simulink model "gm_sampleModel1714_sub"  (R2023a)
settings: Solver=VariableStepAuto  StartTime=0.0  StopTime=10.0  RelTol=1e-3
libraries: simulink x2, hdlsllib x1
settings Model: Creator=user1  LastModifiedBy=user1
settings OptimizationCC: BlockReduction=off  ConditionallyExecuteInputs=off
settings DebuggingCC: InheritedTsInSrcMsg=none

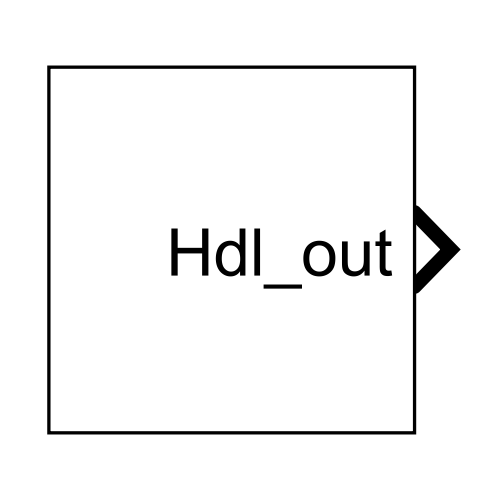
[thumbnail: Simulink's stored preview of the top-level diagram]
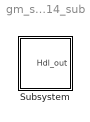
== system gm_sampleModel1714_sub ==
  Subsystem : Subsystem

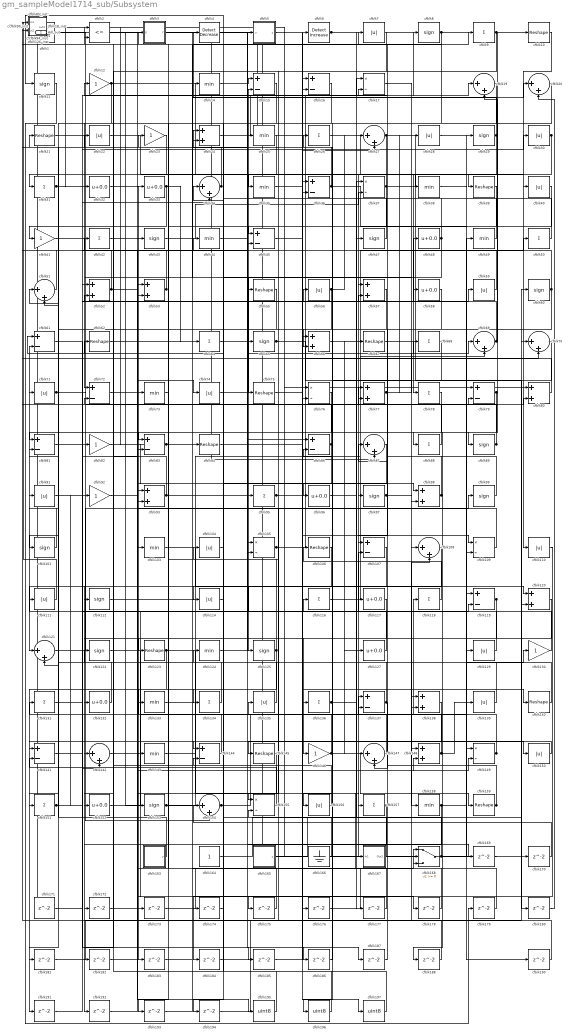
== system gm_sampleModel1714_sub/Subsystem ==
  cfblk1 : hdlsllib/Logic and Bit Operations/Bit Shift  mode=Shift Left Logical  N=0
  cfblk{10,21,39,55,62,67,75,84,106,123,140,145,159} (13 alike) : Reshape
  cfblk{8,11,29,43,47,60,65,89,97,99,101,112,122,125,153} (15 alike) : Signum
  cfblk102_inst : Subsystem
  cfblk{14,25,35,38,44,49,73,103,124,133,143,158} (12 alike) : MinMax  OutDataTypeStr=uint8
  cfblk{7,22,28,30,40,56,59,71,74,91,104,110..111,114,129,135,139,150,156} (19 alike) : Abs  OutDataTypeStr=uint8  SaturateOnIntegerOverflow=off
  cfblk{17,37,76,105,109,149,155} (7 alike) : Product  Inputs=*/  OutDataTypeStr=uint8  RndMeth=Zero  SaturateOnIntegerOverflow=on
  cfblk{15..16,36,45,61,72,79,81,83,86,107,119,137,141,144} (15 alike) : Sum  Inputs=+-  OutDataTypeStr=uint8
  cfblk{19..20,27,34,51,69..70,87,108,121,142,147,154} (13 alike) : Sum  Inputs=|++  OutDataTypeStr=uint8
  cfblk113_inst : Subsystem
  cfblk{9,26,31,42,50,64,68,78,88,95,116,118,131,134,136,151,157} (17 alike) : Sum  Inputs=+  OutDataTypeStr=uint8
  cfblk{32..33,48,58,96,117,127,132,152} (9 alike) : Bias  Bias=0.0  SaturateOnIntegerOverflow=off
  cfblk{12,23,41,82,92,130,146} (7 alike) : Gain  OutDataTypeStr=uint8
  cfblk{24,52..53,57,66,77,80,93,98,120,138,148} (12 alike) : Sum  OutDataTypeStr=uint8
  cfblk126_inst : Subsystem
  cfblk128_inst : Subsystem
  cfblk163 : Subsystem  mask(Counter Free-Running){NumBits=double(16), tsamp=double(-1)}
      mask prompts: NumBits "Simulink:masks:NumberOfBits_MP"; tsamp "Simulink:masks:SampleTime_MP"
      mask help: Simulink:masks:CounterFreeRunning_MD
  cfblk164 : Constant  OutDataTypeStr=uint8  SampleTime=-1
  cfblk165 : Subsystem  mask(Counter Limited){uplimit=double(7), tsamp=double(-1)}
      mask prompts: uplimit "Simulink:masks:UpperLimit_MP"; tsamp "Simulink:masks:SampleTime_MP"
      mask help: Simulink:masks:CounterLimited_MD
      mask init:
      | nbits = double(8);
      | tsamp = double(-1);
      | uplimit = double(7);
  cfblk166 : Ground
  cfblk167 : Subsystem
  cfblk168 : Switch  OutDataTypeStr=uint8  SaturateOnIntegerOverflow=off  InputSameDT=off
  cfblk{169..188,190..194} (25 alike) : Delay  SampleTime=1
  cfblk18_inst : Subsystem
  cfblk195 : DataTypeConversion  OutDataTypeStr=uint8  SaturateOnIntegerOverflow=off  RndMeth=Floor
  cfblk196 : DataTypeConversion  OutDataTypeStr=uint8  SaturateOnIntegerOverflow=off  RndMeth=Floor
  cfblk197 : DataTypeConversion  OutDataTypeStr=uint8  SaturateOnIntegerOverflow=off  RndMeth=Floor
  cfblk2 : RelationalOperator  Operator=<=  OutDataTypeStr=boolean  InputSameDT=off
  cfblk3 : Subsystem  mask(Detect Fall Nonpositive){vinit=double(0), InputProcessing=Elements as channels (sample based), OutDataTypeStr=uint8}
      mask prompts: vinit "Simulink:masks:InitialCondition_MP"; InputProcessing "Simulink:masks:InputProcessing_MP"; OutDataTypeStr "Simulink:masks:OutputDataType_MP"
      mask help: Simulink:masks:DetectFallNonpositive_MD
      mask init:
      | InputProcessing = 'Elements as channels (sample based)';
      | OutDataTypeStr = 'uint8';
      | vinit = double(0);
      mask TypeOptions InputProcessing: Simulink:masks:ColumnsAsChannelsFrameBased | Simulink:masks:ElementsAsChannelsSampleBased
      mask TypeOptions OutDataTypeStr: Simulink:masks:uint8 | Simulink:masks:boolean
      mask Display: fprintf('U <= 0\n&  NOT\nU/z <= 0')
  cfblk4 : simulink/Logic and Bit Operations/Detect Decrease  vinit=0.0  OutDataTypeStr=uint8
      settings: LibrarySourceBlock=|
      | hdlsllib/Logic and Bit
      | Operations/Detect
      | Decrease
  cfblk5 : Subsystem  mask(Compare To Constant){relop=<=, const=double(3), OutDataTypeStr=uint8, ZeroCross=on}
      mask prompts: relop "Simulink:masks:Operator_MP"; const "Simulink:masks:ConstantValue_MP"; OutDataTypeStr "Simulink:masks:OutputDataType_MP"; ZeroCross "Simulink:masks:EnableZerocrossingDetection_MP"
      mask help: Simulink:masks:CompareToConstant_MD
      mask init:
      | OutDataTypeStr = 'uint8';
      | ZeroCross = 'on';
      | blkName = 'sampleModel1714_sub/Subsystem/cfblk5';
      | const = double(3);
      | const_str = '3.0';
      | const_val = double(3);
      | relop = '<=';
      | setValue = 'fixdt(0, 8)';
      | str = '<= 3';
      mask TypeOptions relop: == | ~= | < | <= | >= | >
      mask TypeOptions OutDataTypeStr: Simulink:masks:uint8 | Simulink:masks:boolean
      mask Callback ZeroCross: sl('zeroCrossEnable', gcbh);
      mask Display: disp(str)
  cfblk6 : simulink/Logic and Bit Operations/Detect Increase  vinit=0.0  OutDataTypeStr=uint8
      settings: LibrarySourceBlock=|
      | hdlsllib/Logic and Bit
      | Operations/Detect
      | Increase
  cfblk85_inst : Subsystem
  cfblk90_inst : Subsystem
  cfblk94_inst : Subsystem
  Hdl_out : Outport  OutDataTypeStr=uint8  SampleTime=1
  wires:
  cfblk1/1 -> cfblk154/2
  cfblk10/1 -> cfblk110/1
  cfblk101/1 -> cfblk61/2
  cfblk102_inst/1(out1) -> cfblk84/1
  cfblk103/1 -> cfblk120/1
  cfblk104/1 -> cfblk11/1
  cfblk105/1 -> cfblk80/2, cfblk19/1
  cfblk106/1 -> cfblk192/1
  cfblk107/1 -> cfblk121/1
  cfblk108/1 -> cfblk125/1
  cfblk109/1 -> cfblk33/1
  cfblk11/1 -> cfblk179/1
  cfblk110/1 -> cfblk184/1
  cfblk111/1 -> cfblk126_inst/1(in1)
  cfblk112/1 -> cfblk50/1
  cfblk113_inst/1(out1) -> cfblk87/2, cfblk128_inst/1(in1)
  cfblk114/1 -> cfblk34/1
  cfblk116/1 -> cfblk69/2
  cfblk117/1 -> cfblk146/1
  cfblk118/1 -> cfblk106/1
  cfblk119/1 -> cfblk142/1, cfblk132/1
  cfblk12/1 -> cfblk72/1, cfblk167/1(In1)
  cfblk120/1 -> cfblk136/1
  cfblk121/1 -> cfblk99/1
  cfblk122/1 -> cfblk175/1
  cfblk123/1 -> cfblk168/1, cfblk191/1
  cfblk124/1 -> cfblk86/1
  cfblk125/1 -> cfblk183/1, cfblk3/1(U)
  cfblk126_inst/1(out1) -> cfblk80/1
  cfblk127/1 -> cfblk107/2
  cfblk128_inst/1(out1) -> cfblk171/1
  cfblk129/1 -> cfblk71/1
  cfblk130/1 -> cfblk15/2
  cfblk131/1 -> cfblk116/1
  cfblk132/1 -> cfblk21/1
  cfblk133/1 -> cfblk5/1(u)
  cfblk134/1 -> cfblk81/2
  cfblk135/1 -> cfblk91/1
  cfblk136/1 -> cfblk47/1, cfblk127/1
  cfblk137/1 -> cfblk147/2, cfblk122/1
  cfblk138/1 -> cfblk152/1
  cfblk139/1 -> cfblk87/1
  cfblk14/1 -> cfblk15/1
  cfblk140/1 -> cfblk111/1
  cfblk141/1 -> cfblk30/1
  cfblk142/1 -> cfblk117/1
  cfblk143/1 -> cfblk76/1
  cfblk144/1 -> cfblk52/2
  cfblk145/1 -> cfblk193/1
  cfblk146/1 -> cfblk93/2, cfblk67/1, cfblk159/1
  cfblk147/1 -> cfblk26/1
  cfblk148/1 -> cfblk139/1, cfblk121/2, cfblk95/1
  cfblk149/1 -> cfblk135/1, cfblk118/1, cfblk131/1
  cfblk15/1 -> cfblk134/1
  cfblk150/1 -> cfblk141/1
  cfblk151/1 -> cfblk56/1, cfblk92/1, cfblk17/2
  cfblk152/1 -> cfblk137/1
  cfblk153/1 -> cfblk148/2, cfblk49/1
  cfblk154/1 -> cfblk16/2, Hdl_out/1
  cfblk155/1 -> cfblk141/2
  cfblk156/1 -> cfblk18_inst/1(in1)
  cfblk157/1 -> cfblk173/1, cfblk172/1
  cfblk158/1 -> cfblk194/1, cfblk130/1
  cfblk159/1 -> cfblk85_inst/2(in2), cfblk52/1
  cfblk16/1 -> cfblk153/1
  cfblk163/1(y) -> cfblk51/1
  cfblk164/1 -> cfblk70/1
  cfblk165/1(y) -> cfblk37/1
  cfblk166/1 -> cfblk105/1
  cfblk167/1(Out1) -> cfblk61/1
  cfblk168/1 -> cfblk79/1, cfblk124/1
  cfblk169/1 -> cfblk1/1
  cfblk17/1 -> cfblk148/1
  cfblk170/1 -> cfblk154/1
  cfblk171/1 -> cfblk34/2
  cfblk172/1 -> cfblk45/2
  cfblk173/1 -> cfblk168/2
  cfblk174/1 -> cfblk144/2
  cfblk175/1 -> cfblk24/1
  cfblk176/1 -> cfblk138/1
  cfblk177/1 -> cfblk93/1
  cfblk178/1 -> cfblk16/1
  cfblk179/1 -> cfblk53/1
  cfblk18_inst/1(out1) -> cfblk29/1
  cfblk180/1 -> cfblk20/2
  cfblk181/1 -> cfblk108/2
  cfblk182/1 -> cfblk119/2
  cfblk183/1 -> cfblk168/3
  cfblk184/1 -> cfblk120/2
  cfblk185/1 -> cfblk36/1
  cfblk186/1 -> cfblk86/2
  cfblk187/1 -> cfblk137/2
  cfblk188/1 -> cfblk155/2
  cfblk19/1 -> cfblk41/1
  cfblk190/1 -> cfblk102_inst/2(in2)
  cfblk191/1 -> cfblk142/2
  cfblk192/1 -> cfblk149/2
  cfblk193/1 -> cfblk9/1
  cfblk194/1 -> cfblk60/1
  cfblk195/1 -> cfblk104/1
  cfblk196/1 -> cfblk2/1
  cfblk197/1 -> cfblk2/2
  cfblk2/1 -> cfblk195/1
  cfblk20/1 -> cfblk123/1
  cfblk21/1 -> cfblk75/1
  cfblk22/1 -> cfblk78/1
  cfblk23/1 -> cfblk53/2
  cfblk24/1 -> cfblk8/1
  cfblk25/1 -> cfblk143/1
  cfblk26/1 -> cfblk39/1
  cfblk27/1 -> cfblk181/1, cfblk180/1
  cfblk28/1 -> cfblk190/1
  cfblk29/1 -> cfblk182/1, cfblk4/1
  cfblk3/1(Y) -> cfblk57/1
  cfblk30/1 -> cfblk36/2, cfblk31/1
  cfblk31/1 -> cfblk108/1, cfblk176/1
  cfblk32/1 -> cfblk97/1
  cfblk33/1 -> cfblk51/2, cfblk64/1
  cfblk34/1 -> cfblk126_inst/2(in2), cfblk113_inst/2(in2)
  cfblk35/1 -> cfblk109/1
  cfblk36/1 -> cfblk85_inst/1(in1), cfblk129/1
  cfblk37/1 -> cfblk40/1, cfblk145/1, cfblk35/1
  cfblk38/1 -> cfblk119/1
  cfblk39/1 -> cfblk155/1
  cfblk4/1 -> cfblk98/1
  cfblk40/1 -> cfblk83/1
  cfblk41/1 -> cfblk73/1
  cfblk42/1 -> cfblk103/1
  cfblk43/1 -> cfblk37/2
  cfblk44/1 -> cfblk186/1
  cfblk45/1 -> cfblk6/1
  cfblk47/1 -> cfblk23/1
  cfblk48/1 -> cfblk24/2, cfblk76/2, cfblk174/1
  cfblk49/1 -> cfblk7/1
  cfblk5/1(y) -> cfblk157/1
  cfblk50/1 -> cfblk22/1
  cfblk51/1 -> cfblk94_inst/1(in1)
  cfblk52/1 -> cfblk74/1, cfblk42/1
  cfblk53/1 -> cfblk90_inst/2(in2), cfblk102_inst/1(in1)
  cfblk55/1 -> cfblk114/1
  cfblk56/1 -> cfblk81/1, cfblk27/1
  cfblk57/1 -> cfblk156/1
  cfblk58/1 -> cfblk107/1
  cfblk59/1 -> cfblk90_inst/1(in1)
  cfblk6/1 -> cfblk147/1, cfblk38/1
  cfblk60/1 -> cfblk65/1, cfblk113_inst/1(in1)
  cfblk61/1 -> cfblk82/1
  cfblk62/1 -> cfblk20/1
  cfblk64/1 -> cfblk150/1
  cfblk65/1 -> cfblk70/2, cfblk158/1
  cfblk66/1 -> cfblk138/2
  cfblk67/1 -> cfblk149/1
  cfblk68/1 -> cfblk96/1
  cfblk69/1 -> cfblk57/2, cfblk48/1, cfblk19/2
  cfblk7/1 -> cfblk45/1
  cfblk70/1 -> cfblk98/2
  cfblk71/1 -> cfblk79/2, cfblk14/1, cfblk44/1
  cfblk72/1 -> cfblk178/1
  cfblk73/1 -> cfblk133/1
  cfblk74/1 -> cfblk68/1
  cfblk75/1 -> cfblk140/1
  cfblk76/1 -> cfblk101/1
  cfblk77/1 -> cfblk69/1, cfblk28/1
  cfblk78/1 -> cfblk196/1
  cfblk79/1 -> cfblk188/1, cfblk151/1
  cfblk8/1 -> cfblk66/2, cfblk128_inst/2(in2)
  cfblk80/1 -> cfblk94_inst/2(in2)
  cfblk81/1 -> cfblk185/1
  cfblk82/1 -> cfblk177/1
  cfblk83/1 -> cfblk59/1, cfblk25/1
  cfblk84/1 -> cfblk77/1
  cfblk85_inst/1(out1) -> cfblk10/1
  cfblk86/1 -> cfblk72/2, cfblk18_inst/2(in2), cfblk144/1
  cfblk87/1 -> cfblk105/2
  cfblk88/1 -> cfblk66/1
  cfblk89/1 -> cfblk43/1, cfblk88/1
  cfblk9/1 -> cfblk89/1, cfblk112/1
  cfblk90_inst/1(out1) -> cfblk32/1
  cfblk91/1 -> cfblk83/2
  cfblk92/1 -> cfblk187/1
  cfblk93/1 -> cfblk62/1, cfblk169/1
  cfblk94_inst/1(out1) -> cfblk170/1
  cfblk95/1 -> cfblk27/2, cfblk197/1
  cfblk96/1 -> cfblk58/1
  cfblk97/1 -> cfblk77/2, cfblk109/2
  cfblk98/1 -> cfblk17/1, cfblk12/1
  cfblk99/1 -> cfblk55/1

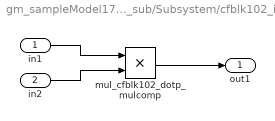
== system gm_sampleModel1714_sub/Subsystem/cfblk102_inst ==
  in1 : Inport  OutDataTypeStr=uint8  SampleTime=1
  in2 : Inport  Port=2  OutDataTypeStr=uint8  SampleTime=1
  mul_cfblk102_dotp_mulcomp : Product  Inputs=**  OutDataTypeStr=uint8  SampleTime=1
  out1 : Outport  OutDataTypeStr=uint8  SampleTime=1
  wires:
  in1/1 -> mul_cfblk102_dotp_mulcomp/1
  in2/1 -> mul_cfblk102_dotp_mulcomp/2
  mul_cfblk102_dotp_mulcomp/1 -> out1/1

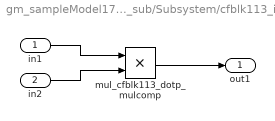
== system gm_sampleModel1714_sub/Subsystem/cfblk113_inst ==
  in1 : Inport  OutDataTypeStr=uint8  SampleTime=1
  in2 : Inport  Port=2  OutDataTypeStr=uint8  SampleTime=1
  mul_cfblk113_dotp_mulcomp : Product  Inputs=**  OutDataTypeStr=uint8  SampleTime=1
  out1 : Outport  OutDataTypeStr=uint8  SampleTime=1
  wires:
  in1/1 -> mul_cfblk113_dotp_mulcomp/1
  in2/1 -> mul_cfblk113_dotp_mulcomp/2
  mul_cfblk113_dotp_mulcomp/1 -> out1/1

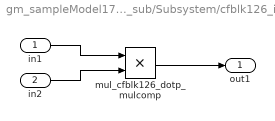
== system gm_sampleModel1714_sub/Subsystem/cfblk126_inst ==
  in1 : Inport  OutDataTypeStr=uint8  SampleTime=1
  in2 : Inport  Port=2  OutDataTypeStr=uint8  SampleTime=1
  mul_cfblk126_dotp_mulcomp : Product  Inputs=**  OutDataTypeStr=uint8  SampleTime=1
  out1 : Outport  OutDataTypeStr=uint8  SampleTime=1
  wires:
  in1/1 -> mul_cfblk126_dotp_mulcomp/1
  in2/1 -> mul_cfblk126_dotp_mulcomp/2
  mul_cfblk126_dotp_mulcomp/1 -> out1/1

== system gm_sampleModel1714_sub/Subsystem/cfblk128_inst ==
  in1 : Inport  OutDataTypeStr=uint8  SampleTime=1
  in2 : Inport  Port=2  OutDataTypeStr=uint8  SampleTime=1
  mul_cfblk128_dotp_mulcomp : Product  Inputs=**  OutDataTypeStr=uint8  SampleTime=1
  out1 : Outport  OutDataTypeStr=uint8  SampleTime=1
  wires:
  in1/1 -> mul_cfblk128_dotp_mulcomp/1
  in2/1 -> mul_cfblk128_dotp_mulcomp/2
  mul_cfblk128_dotp_mulcomp/1 -> out1/1

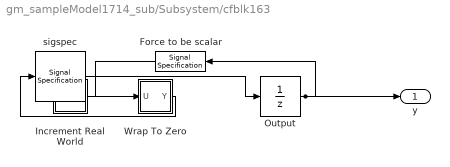
== system gm_sampleModel1714_sub/Subsystem/cfblk163 ==
  Force to be scalar : SignalSpecification  DisableCoverage=on  Dimensions=1
  Increment Real World : Subsystem  mask(Real World Value Increment){}
      mask help: Simulink:masks:RealWorldValueIncrement_MD
      mask Display: disp('V++')
  Output : UnitDelay  InitialCondition=0.0  SampleTime=tsamp  HasFrameUpgradeWarning=on
  Wrap To Zero : Subsystem  mask(Wrap To Zero){Threshold=double(65535)}
      mask prompts: Threshold "Simulink:masks:Threshold_MP"
      mask help: Simulink:masks:WrapToZero_MD
  sigspec : SignalSpecification  OutDataTypeStr=uint16  Dimensions=1
  y : Outport  SampleTime=1
  wires:
  Force to be scalar/1 -> Increment Real World/1(u)
  Increment Real World/1(y) -> Wrap To Zero/1(U)
  Output/1 -> Force to be scalar/1, y/1
  Wrap To Zero/1(Y) -> sigspec/1
  sigspec/1 -> Output/1

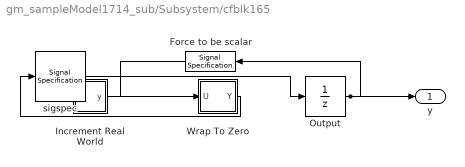
== system gm_sampleModel1714_sub/Subsystem/cfblk165 ==
  Force to be scalar : SignalSpecification  DisableCoverage=on  Dimensions=1
  Increment Real World : Subsystem  mask(Real World Value Increment){}
      mask help: Simulink:masks:RealWorldValueIncrement_MD
      mask Display: disp('V++')
  Output : UnitDelay  InitialCondition=0.0  SampleTime=tsamp  HasFrameUpgradeWarning=on
  Wrap To Zero : Subsystem  mask(Wrap To Zero){Threshold=double(7)}
      mask prompts: Threshold "Simulink:masks:Threshold_MP"
      mask help: Simulink:masks:WrapToZero_MD
  sigspec : SignalSpecification  OutDataTypeStr=uint8  Dimensions=1
  y : Outport  SampleTime=1
  wires:
  Force to be scalar/1 -> Increment Real World/1(u)
  Increment Real World/1(y) -> Wrap To Zero/1(U)
  Output/1 -> Force to be scalar/1, y/1
  Wrap To Zero/1(Y) -> sigspec/1
  sigspec/1 -> Output/1

== system gm_sampleModel1714_sub/Subsystem/cfblk167 ==
  In1 : Inport  OutDataTypeStr=uint8  PortDimensions=1  SampleTime=1
  Out1 : Outport  SampleTime=1
  wires:
  In1/1 -> Out1/1

== system gm_sampleModel1714_sub/Subsystem/cfblk18_inst ==
  in1 : Inport  OutDataTypeStr=uint8  SampleTime=1
  in2 : Inport  Port=2  OutDataTypeStr=uint8  SampleTime=1
  mul_cfblk18_dotp_mulcomp : Product  Inputs=**  OutDataTypeStr=uint8  SampleTime=1
  out1 : Outport  OutDataTypeStr=uint8  SampleTime=1
  wires:
  in1/1 -> mul_cfblk18_dotp_mulcomp/1
  in2/1 -> mul_cfblk18_dotp_mulcomp/2
  mul_cfblk18_dotp_mulcomp/1 -> out1/1

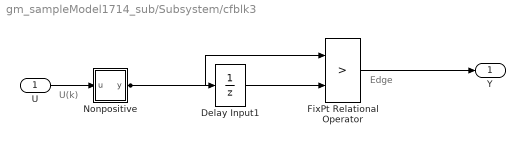
== system gm_sampleModel1714_sub/Subsystem/cfblk3 ==
  note: U(k)
  note: Edge
  U : Inport  OutDataTypeStr=uint8  SampleTime=1
  Delay Input1 : UnitDelay  Description=Store in Global RAM  DisableCoverage=on  InitialCondition=vinit  SampleTime=-1  HasFrameUpgradeWarning=on
  FixPt Relational Operator : RelationalOperator  Operator=>  OutDataTypeStr=fixdt(0, 8)  ZeroCross=off  InputSameDT=off
  Nonpositive : Subsystem  mask(Compare To Zero){relop=<=, OutDataTypeStr=boolean, ZeroCross=off}
      mask prompts: relop "Simulink:masks:Operator_MP"; OutDataTypeStr "Simulink:masks:OutputDataType_MP"; ZeroCross "Simulink:masks:EnableZerocrossingDetection_MP"
      mask help: Simulink:masks:CompareToZero_MD
      mask init:
      | OutDataTypeStr = 'boolean';
      | ZeroCross = 'off';
      | blkName = 'sampleModel1714_sub/Subsystem/cfblk3/Nonpositive';
      | relop = '<=';
      | setValue = 'boolean';
      mask TypeOptions relop: == | ~= | < | <= | >= | >
      mask TypeOptions OutDataTypeStr: Simulink:masks:uint8 | Simulink:masks:boolean
      mask Callback ZeroCross: sl('zeroCrossEnable', gcbh);
      mask Display: disp([relop,' 0'])
  Y : Outport  SampleTime=1
  wires:
  U/1 -> Nonpositive/1(u)
  Delay Input1/1 -> FixPt Relational Operator/2
  FixPt Relational Operator/1 -> Y/1
  Nonpositive/1(y) -> FixPt Relational Operator/1, Delay Input1/1

== system gm_sampleModel1714_sub/Subsystem/cfblk5 ==
  u : Inport  OutDataTypeStr=uint8  SampleTime=1
  Compare : RelationalOperator  Operator=<=  OutDataTypeStr=fixdt(0, 8)
  Constant : Constant  DisableCoverage=on  Value=const  OutDataTypeStr=Inherit: Inherit via back propagation  SampleTime=-1
  y : Outport  SampleTime=1
  wires:
  u/1 -> Compare/1
  Compare/1 -> y/1
  Constant/1 -> Compare/2

== system gm_sampleModel1714_sub/Subsystem/cfblk85_inst ==
  in1 : Inport  OutDataTypeStr=uint8  SampleTime=1
  in2 : Inport  Port=2  OutDataTypeStr=uint8  SampleTime=1
  mul_cfblk85_dotp_mulcomp : Product  Inputs=**  OutDataTypeStr=uint8  SampleTime=1
  out1 : Outport  OutDataTypeStr=uint8  SampleTime=1
  wires:
  in1/1 -> mul_cfblk85_dotp_mulcomp/1
  in2/1 -> mul_cfblk85_dotp_mulcomp/2
  mul_cfblk85_dotp_mulcomp/1 -> out1/1

== system gm_sampleModel1714_sub/Subsystem/cfblk90_inst ==
  in1 : Inport  OutDataTypeStr=uint8  SampleTime=1
  in2 : Inport  Port=2  OutDataTypeStr=uint8  SampleTime=1
  mul_cfblk90_dotp_mulcomp : Product  Inputs=**  OutDataTypeStr=uint8  SampleTime=1
  out1 : Outport  OutDataTypeStr=uint8  SampleTime=1
  wires:
  in1/1 -> mul_cfblk90_dotp_mulcomp/1
  in2/1 -> mul_cfblk90_dotp_mulcomp/2
  mul_cfblk90_dotp_mulcomp/1 -> out1/1

== system gm_sampleModel1714_sub/Subsystem/cfblk94_inst ==
  in1 : Inport  OutDataTypeStr=uint8  SampleTime=1
  in2 : Inport  Port=2  OutDataTypeStr=uint8  SampleTime=1
  mul_cfblk94_dotp_mulcomp : Product  Inputs=**  OutDataTypeStr=uint8  SampleTime=1
  out1 : Outport  OutDataTypeStr=uint8  SampleTime=1
  wires:
  in1/1 -> mul_cfblk94_dotp_mulcomp/1
  in2/1 -> mul_cfblk94_dotp_mulcomp/2
  mul_cfblk94_dotp_mulcomp/1 -> out1/1

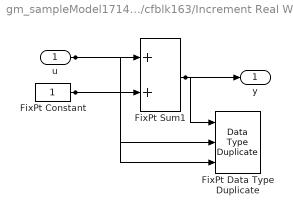
== system gm_sampleModel1714_sub/Subsystem/cfblk163/Increment Real World ==
  u : Inport  OutDataTypeStr=uint16  SampleTime=1
  FixPt Constant : Constant  DisableCoverage=on  OutDataTypeStr=Inherit: Inherit via back propagation  SampleTime=-1
  FixPt Data Type Duplicate : DataTypeDuplicate  DisableCoverage=on  NumInputPorts=3
  FixPt Sum1 : Sum  InputSameDT=on  OutDataTypeStr=Inherit: Inherit via back propagation  LockScale=on
  y : Outport  SampleTime=1
  wires:
  u/1 -> FixPt Sum1/1, FixPt Data Type Duplicate/2
  FixPt Constant/1 -> FixPt Sum1/2, FixPt Data Type Duplicate/3
  FixPt Sum1/1 -> FixPt Data Type Duplicate/1, y/1

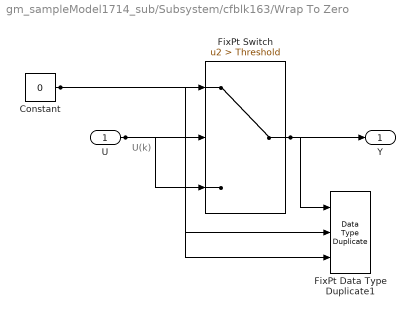
== system gm_sampleModel1714_sub/Subsystem/cfblk163/Wrap To Zero ==
  note: U(k)
  U : Inport  OutDataTypeStr=uint16  SampleTime=1
  Constant : Constant  DisableCoverage=on  Value=0  OutDataTypeStr=Inherit: Inherit via back propagation  SampleTime=-1
  FixPt Data Type Duplicate1 : DataTypeDuplicate  DisableCoverage=on  NumInputPorts=3
  FixPt Switch : Switch  Criteria=u2 > Threshold  Threshold=Threshold  OutDataTypeStr=Inherit: Inherit via back propagation  ZeroCross=off  SaturateOnIntegerOverflow=off  InputSameDT=off
  Y : Outport  SampleTime=1
  wires:
  U/1 -> FixPt Switch/3, FixPt Switch/2, FixPt Data Type Duplicate1/2
  Constant/1 -> FixPt Switch/1, FixPt Data Type Duplicate1/3
  FixPt Switch/1 -> FixPt Data Type Duplicate1/1, Y/1

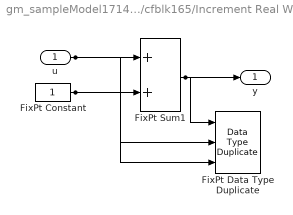
== system gm_sampleModel1714_sub/Subsystem/cfblk165/Increment Real World ==
  u : Inport  OutDataTypeStr=uint8  SampleTime=1
  FixPt Constant : Constant  DisableCoverage=on  OutDataTypeStr=Inherit: Inherit via back propagation  SampleTime=-1
  FixPt Data Type Duplicate : DataTypeDuplicate  DisableCoverage=on  NumInputPorts=3
  FixPt Sum1 : Sum  InputSameDT=on  OutDataTypeStr=Inherit: Inherit via back propagation  LockScale=on
  y : Outport  SampleTime=1
  wires:
  u/1 -> FixPt Sum1/1, FixPt Data Type Duplicate/2
  FixPt Constant/1 -> FixPt Sum1/2, FixPt Data Type Duplicate/3
  FixPt Sum1/1 -> FixPt Data Type Duplicate/1, y/1

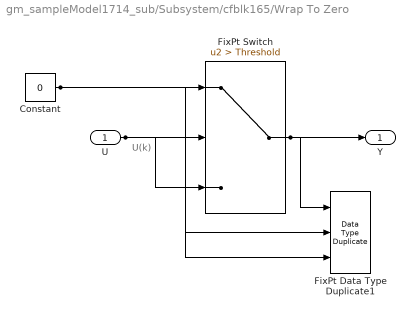
== system gm_sampleModel1714_sub/Subsystem/cfblk165/Wrap To Zero ==
  note: U(k)
  U : Inport  OutDataTypeStr=uint8  SampleTime=1
  Constant : Constant  DisableCoverage=on  Value=0  OutDataTypeStr=Inherit: Inherit via back propagation  SampleTime=-1
  FixPt Data Type Duplicate1 : DataTypeDuplicate  DisableCoverage=on  NumInputPorts=3
  FixPt Switch : Switch  Criteria=u2 > Threshold  Threshold=Threshold  OutDataTypeStr=Inherit: Inherit via back propagation  ZeroCross=off  SaturateOnIntegerOverflow=off  InputSameDT=off
  Y : Outport  SampleTime=1
  wires:
  U/1 -> FixPt Switch/3, FixPt Switch/2, FixPt Data Type Duplicate1/2
  Constant/1 -> FixPt Switch/1, FixPt Data Type Duplicate1/3
  FixPt Switch/1 -> FixPt Data Type Duplicate1/1, Y/1

== system gm_sampleModel1714_sub/Subsystem/cfblk3/Nonpositive ==
  u : Inport  OutDataTypeStr=uint8  SampleTime=1
  Compare : RelationalOperator  Operator=<=  OutDataTypeStr=boolean  ZeroCross=off
  Constant : Constant  DisableCoverage=on  Value=0  OutDataTypeStr=Inherit: Inherit via back propagation  SampleTime=-1  PreserveConstantTs=on
  y : Outport  SampleTime=1
  wires:
  u/1 -> Compare/1
  Compare/1 -> y/1
  Constant/1 -> Compare/2
